simulink model "AmplitudeModulation"  (R2014b)
settings: Solver=ode45  StartTime=0.0  StopTime=1e-1  MaxStep=1/50000  RelTol=1e-3
settings Model: CovSFcnEnable=on  Creator=baran_000  LastModifiedBy=baran_000
settings OptimizationCC: UseDivisionForNetSlopeComputation=off  SimCompilerOptimization=off
settings DebuggingCC: SolverPrmCheckMsg=none  FrameProcessingCompatibilityMsg=error
settings RTWCC: RTWCompilerOptimization=off

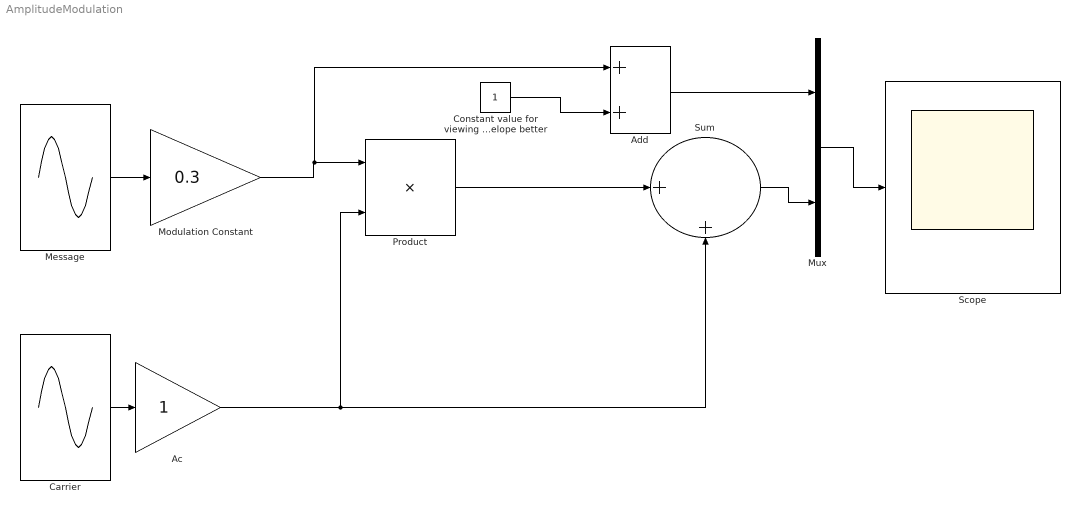
== system AmplitudeModulation ==
  "Ac " : Gain
  Add : Sum
  "Carrier " : Sin  Frequency=2*pi*1000  Phase=pi/2  SampleTime=0
  Constant value for viewing envelope better : Constant
  "Message " : Sin  Frequency=2*pi*100  Phase=pi/2  SampleTime=0
  "Modulation Constant " : Gain  Gain=0.3
  Mux : Mux  Inputs=2
  Product : Product
  Scope : Scope
  Sum : Sum  Inputs=|++
  wires:
  "Message "/1 -> "Modulation Constant "/1
  "Carrier "/1 -> "Ac "/1
  "Ac "/1 -> Product/2, Sum/2
  "Modulation Constant "/1 -> Add/1, Product/1
  Product/1 -> Sum/1
  Sum/1 -> Mux/2
  Mux/1 -> Scope/1
  Constant value for viewing envelope better/1 -> Add/2
  Add/1 -> Mux/1
